simulink model "vr_octavia_mirror"  (Simulink 7.7)
settings: Solver=VariableStepDiscrete  StartTime=0.0  StopTime=111.56  RelTol=1e-3
PostLoadFcn:
  | load octavia_testlap
libraries: vrlib x26, simulink x1
Description:
  | Vehicle Dynamics Visualization with Live Rear Mirror Image
  | 
  | This example extends the vr_octavia example to demonstrate the capability
  | of the VR Sink block to process video stream on input.
  | 
  | In the virtual world, a VRML97 PixelTexture texture map is defined
  | at the place of the vehicle left rear mirror. 2D image from a viewpoint placed
  | at the same position (looking backwards) is mirrored and looped back into
  | the same virtual world and projected on the rear mirror glass - creating
  | an impression of live reflection.
  | 
  | Texture image can have different formats (corresponding to the available
  | SFImage definitions according to the VRML97 standard), in this case
  | we use an RGB image that has the same format as the output from the
  | VR to Video block. Note that in the VRML file associated with the scene,
  | it is possible to define only a trivial texture (in our case, a 4x4 pixel
  | checkerboard) that will get resized during simulation according to the current
  | size of the signal on the input.
settings Model: Creator=Danek  LastModifiedBy=Danek  ExtModeArmWhenConnect=off  BufferReuse=off
settings SolverCC: InsertRTBMode=Auto
settings DataIOCC: SignalLoggingName=sigsOut
settings OptimizationCC: BooleanDataType=off  InlineInvariantSignals=on  OptimizeBlockIOStorage=off  BufferReuse=off  ExpressionFolding=off  LocalBlockOutputs=off  InitFltsAndDblsToZero=on
settings DebuggingCC: CheckExecutionContextPreStartOutputMsg=on  CheckExecutionContextRuntimeOutputMsg=on  SignalResolutionControl=TryResolveAllWithWarning  SolverPrmCheckMsg=none  MultiTaskDSMMsg=warning  MultiTaskCondExecSysMsg=none  StrictBusMsg=None
settings RTWCC: RetainRTWFile=on  ProcessScript=grt_make_rtw_hook  IncludeERTFirstTime=on
settings GRTTargetCC: TargetFcnLib=ansi_tfl_tmw.mat

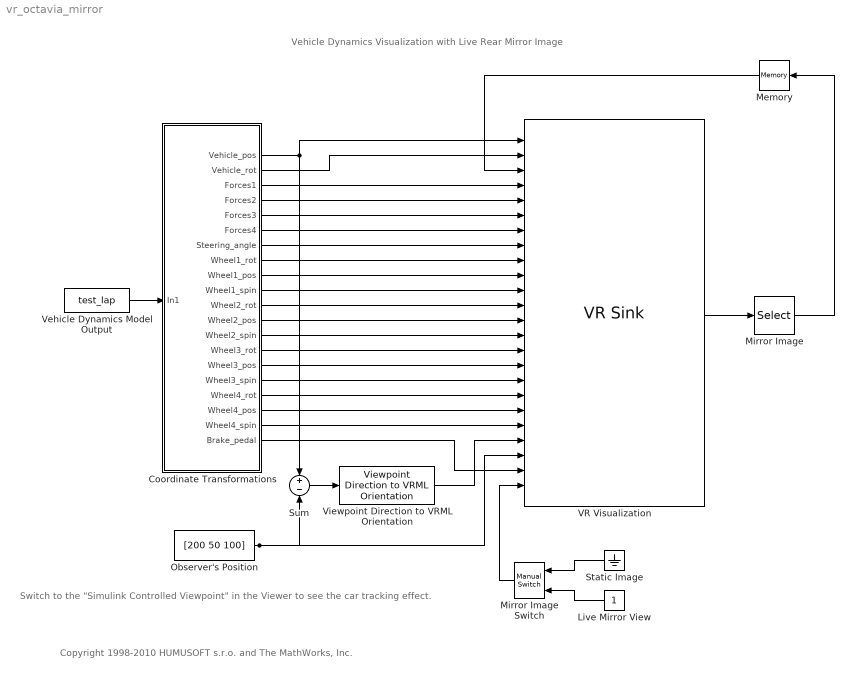
== system vr_octavia_mirror ==
  note: Vehicle Dynamics Visualization with Live Rear Mirror Image
  note: Switch to the "Simulink Controlled Viewpoint"
      | in the Viewer to see the car tracking effect.
  note: Copyright 1998-2010 HUMUSOFT s.r.o. and The MathWorks, Inc.
  Coordinate Transformations : Subsystem
  Live Mirror View : Constant
  Memory : Memory
  Mirror Image : Selector  NumberOfDimensions=3  InputPortWidth=3  IndexOptions=Select all,Index vector (dialog),Select all  Indices=200:-1:1,160:-1:1,1  OutputSizes=1,1,1
  Mirror Image Switch : simulink/Signal Routing/Manual Switch  SystemSampleTime=-1  sw=0  action=0  varsize=off
  Observer's Position : Constant  Value=[200 50 100]
  Static Image : Ground
  Sum : Sum  Inputs=+-
  VR Visualization : vrlib/VR Sink  InstantiateOnLoad=on  SampleTime=0.1  ViewEnable=on  RemoteChange=off  RemoteView=on  FieldsWritten=Vehicle_pos_Car1.translation.3.1.1.double#Vehicle_rot_Car1.rotation.4.1.1.double#Mirror_Image_Car1.image.-1.-1.-1.uint8#Force1_Car1.scale.3.1.1.double#Force2_Car1.scale.3.1.1.double#Force3_Car1.scale.3.1.1.double#Force4_Car1.scale.3.1.1.double#SteeringWheelAngle1_Car1.rotation.4.1.1.double#WheelFL_Car1.rotation.4.1.1.double#WheelFL_Car1.translation.3.1.1.double#WheelSpinFL_Car1.rotation.4.1.1.double#WheelFR_Car1.rotation.4.1.1.double#WheelFR_Car1.translation.3.1.1.double#WheelSpinFR_Car1.rotation.4.1.1.double#WheelRL_Car1.rotation.4.1.1.double#WheelRL_Car1.translation.3.1.1.double#WheelSpinRL_Car1.rotation.4.1.1.double#WheelRR_Car1.rotation.4.1.1.double#WheelRR_Car1.translation.3.1.1.double#WheelSpinRR_Car1.rotation.4.1.1.double#FlyingCamera.orientation.4.1.1.double#FlyingCamera.position.3.1.1.double#Brake_Switch_Car1.whichChoice.1.1.1.double#Mirror_Switch_Car1.whichChoice.1.1.1.double  WorldFileName=octavia_scene.wrl  WorldDescription=Vehicle Dynamics Visualization - Skoda Octavia  AutoView=on  VideoDimensions=[100 160]  FigureProperties="{'Position', 'Name', 'Viewpoint', 'CameraBound', 'CameraDirection', 'CameraPosition', 'CameraUpVector', 'ZoomFactor', 'Antialiasing', 'Headlight', 'Lighting', 'NavPanel', 'StatusBar', 'ToolBar', 'Textures', 'Transparency', 'Wireframe', 'NavZones', 'NavMode', 'NavSpeed', 'Record2DCompressMethod', 'Record2DCompressQuality', 'Record2D', 'Record2DFileName', 'Record2DFPS'; [1.9000000000000000e+001  8.9000000000000000e+001  5.7600000000000000e+002  3.8000000000000000e+002], 'Vehicle Dynamics Visualization - Skoda Octavia', 'Driver''s View - Car1', 'on', [0.0000000000000000e+000  0.0000000000000000e+000 -1.0000000000000000e+000], [0.0000000000000000e+000  0.0000000000000000e+000  0.0000000000000000e+000], [0.0000000000000000e+000  1.0000000000000000e+000  0.0000000000000000e+000], [1.0000000000000000e+000], 'on', 'off', 'on', 'halfbar', 'on', 'on', 'on', 'on', 'off', 'off', 'walk', 'normal', 'auto', [7.5000000000000000e+001], 'off', '%f_anim_%n.avi', [1.5000000000000000e+001]; [6.0000000000000000e+002  6.0000000000000000e+001  1.6000000000000000e+002  1.0000000000000000e+002], 'Vehicle Dynamics Visualization - Skoda Octavia', 'Car1 - View from Above Ahead - Rot', 'on', [5.8249750547694490e-001  5.2158739247318453e-001 -6.2341258258569376e-001], [8.0602203932287431e-001  7.6180911249256611e-001 -8.8299607282409376e+000], [6.8248003830141860e-002  7.3287086238403754e-001  6.7693611887805349e-001], [7.5131480090157765e-001], 'on', 'off', 'on', 'none', 'off', 'off', 'on', 'on', 'off', 'off', 'walk', 'veryslow', 'auto', [7.5000000000000000e+001], 'off', '***video***', [1.5000000000000000e+001]}"
  Vehicle Dynamics Model Output : FromWorkspace  VariableName=test_lap  SampleTime=0.04  OutputAfterFinalValue=Holding final value
  Viewpoint Direction to VRML Orientation : vrlib/Utilities/Viewpoint Direction to VRML Orientation  SystemSampleTime=-1
  wires:
  Vehicle Dynamics Model Output/1 -> Coordinate Transformations/1(In1)
  Sum/1 -> Viewpoint Direction to VRML Orientation/1
  Observer's Position/1 -> Sum/2, VR Visualization/22
  VR Visualization/1 -> Mirror Image/1
  Mirror Image/1 -> Memory/1
  Coordinate Transformations/1(Vehicle_pos) -> Sum/1, VR Visualization/1
  Static Image/1 -> Mirror Image Switch/1
  Live Mirror View/1 -> Mirror Image Switch/2
  Coordinate Transformations/2(Vehicle_rot) -> VR Visualization/2
  Memory/1 -> VR Visualization/3
  Coordinate Transformations/3(Forces1) -> VR Visualization/4
  Coordinate Transformations/4(Forces2) -> VR Visualization/5
  Coordinate Transformations/5(Forces3) -> VR Visualization/6
  Coordinate Transformations/6(Forces4) -> VR Visualization/7
  Coordinate Transformations/7(Steering_angle) -> VR Visualization/8
  Coordinate Transformations/8(Wheel1_rot) -> VR Visualization/9
  Coordinate Transformations/9(Wheel1_pos) -> VR Visualization/10
  Coordinate Transformations/10(Wheel1_spin) -> VR Visualization/11
  Coordinate Transformations/11(Wheel2_rot) -> VR Visualization/12
  Coordinate Transformations/12(Wheel2_pos) -> VR Visualization/13
  Coordinate Transformations/13(Wheel2_spin) -> VR Visualization/14
  Coordinate Transformations/14(Wheel3_rot) -> VR Visualization/15
  Coordinate Transformations/15(Wheel3_pos) -> VR Visualization/16
  Coordinate Transformations/16(Wheel3_spin) -> VR Visualization/17
  Coordinate Transformations/17(Wheel4_rot) -> VR Visualization/18
  Coordinate Transformations/18(Wheel4_pos) -> VR Visualization/19
  Coordinate Transformations/19(Wheel4_spin) -> VR Visualization/20
  Viewpoint Direction to VRML Orientation/1 -> VR Visualization/21
  Coordinate Transformations/20(Brake_pedal) -> VR Visualization/23
  Mirror Image Switch/1 -> VR Visualization/24

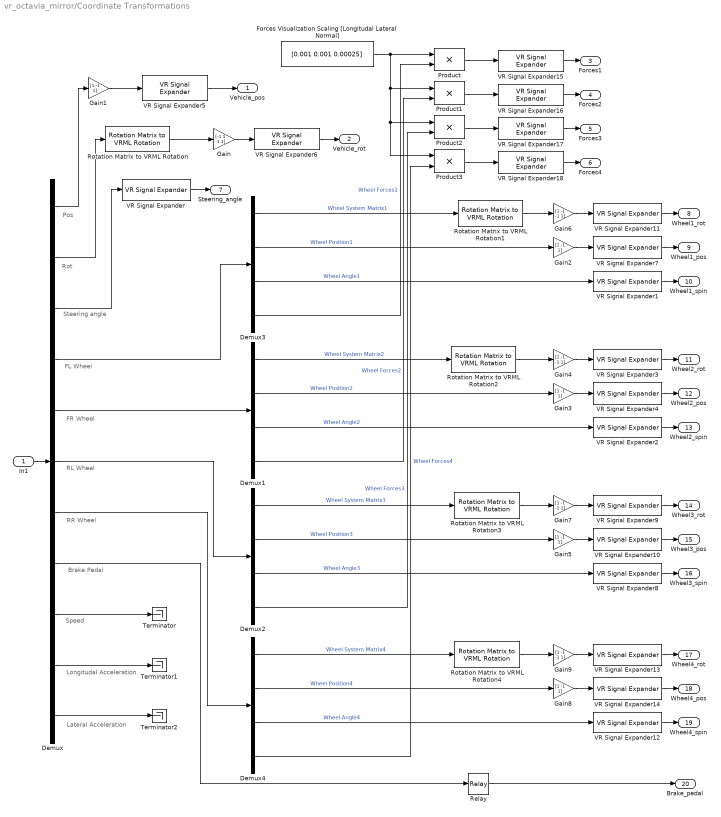
== system vr_octavia_mirror/Coordinate Transformations ==
  note: Steering angle
  note: FL Wheel
  note: FR Wheel
  note: RL Wheel
  note: RR Wheel
  note: Brake Pedal
  note: Pos
  note: Rot
  note: Speed
  note: Longitudal Acceleration
  note: Lateral Acceleration
  In1 : Inport
  Demux : Demux  Outputs=[3,9,1,16,16,16,16,1,1,1,1]
  Demux{1..4} (4 alike) : Demux  Outputs=[9,3,1,3]
  Forces Visualization Scaling [Longitudal Lateral Normal] : Constant  Value=[0.001 0.001 0.00025]
  Gain : Gain  Gain=[-1 1 -1 1]  SaturateOnIntegerOverflow=on  OutDataTypeStr=Inherit: Same as input  ParamDataTypeStr=Inherit: Same as input
  Gain{1..3,5,8} (5 alike) : Gain  Gain=[1 -1 1]  SaturateOnIntegerOverflow=on  OutDataTypeStr=Inherit: Same as input  ParamDataTypeStr=Inherit: Same as input
  Gain{4,6..7,9} (4 alike) : Gain  Gain=[1 -1 -1 1]  SaturateOnIntegerOverflow=on  OutDataTypeStr=Inherit: Same as input  ParamDataTypeStr=Inherit: Same as input
  Product{,1..3} (4 alike) : Product  SaturateOnIntegerOverflow=on  OutDataTypeStr=Inherit: Same as first input
  Relay : Relay
  Rotation Matrix to VRML Rotation{,1..4} (5 alike) : vrlib/Utilities/Rotation Matrix to VRML Rotation  SystemSampleTime=-1  maxzero=1e-12
  Terminator : Terminator
  Terminator1 : Terminator
  Terminator2 : Terminator
  VR Signal Expander{,1..2,8,12} (5 alike) : vrlib/VR Signal Expander  SystemSampleTime=-1  outwidth=4  outidx=[4]
  VR Signal Expander{4,7,10,14} (4 alike) : vrlib/VR Signal Expander  SystemSampleTime=-1  outwidth=3  outidx=[1 3 2 ]
  VR Signal Expander{3,6,9,11,13} (5 alike) : vrlib/VR Signal Expander  SystemSampleTime=-1  outwidth=4  outidx=[1 3 2 4]
  VR Signal Expander{5,15..18} (5 alike) : vrlib/VR Signal Expander  SystemSampleTime=-1  outwidth=3  outidx=[1 3 2]
  Vehicle_pos : Outport
  Vehicle_rot : Outport  Port=2
  Forces1 : Outport  Port=3
  Forces2 : Outport  Port=4
  Forces3 : Outport  Port=5
  Forces4 : Outport  Port=6
  Steering_angle : Outport  Port=7
  Wheel1_rot : Outport  Port=8
  Wheel1_pos : Outport  Port=9
  Wheel1_spin : Outport  Port=10
  Wheel2_rot : Outport  Port=11
  Wheel2_pos : Outport  Port=12
  Wheel2_spin : Outport  Port=13
  Wheel3_rot : Outport  Port=14
  Wheel3_pos : Outport  Port=15
  Wheel3_spin : Outport  Port=16
  Wheel4_rot : Outport  Port=17
  Wheel4_pos : Outport  Port=18
  Wheel4_spin : Outport  Port=19
  Brake_pedal : Outport  Port=20
  wires:
  Gain1/1 -> VR Signal Expander5/1
  Rotation Matrix to VRML Rotation/1 -> Gain/1
  Gain/1 -> VR Signal Expander6/1
  Gain6/1 -> VR Signal Expander11/1
  Gain2/1 -> VR Signal Expander7/1
  Demux3/1 -> Rotation Matrix to VRML Rotation1/1  "Wheel System Matrix1"
  Demux3/2 -> Gain2/1  "Wheel Position1"
  Demux3/3 -> VR Signal Expander1/1  "Wheel Angle1"
  Gain4/1 -> VR Signal Expander3/1
  Rotation Matrix to VRML Rotation2/1 -> Gain4/1
  Gain3/1 -> VR Signal Expander4/1
  Demux1/1 -> Rotation Matrix to VRML Rotation2/1  "Wheel System Matrix2"
  Demux1/2 -> Gain3/1  "Wheel Position2"
  Demux1/3 -> VR Signal Expander2/1  "Wheel Angle2"
  Gain7/1 -> VR Signal Expander9/1
  Rotation Matrix to VRML Rotation3/1 -> Gain7/1
  Demux2/4 -> Product2/2  "Wheel Forces3"
  Gain5/1 -> VR Signal Expander10/1
  Demux2/1 -> Rotation Matrix to VRML Rotation3/1  "Wheel System Matrix3"
  Demux2/2 -> Gain5/1  "Wheel Position3"
  Demux2/3 -> VR Signal Expander8/1  "Wheel Angle3"
  Gain9/1 -> VR Signal Expander13/1
  Rotation Matrix to VRML Rotation4/1 -> Gain9/1
  Demux4/4 -> Product3/2  "Wheel Forces4"
  Gain8/1 -> VR Signal Expander14/1
  Demux4/1 -> Rotation Matrix to VRML Rotation4/1  "Wheel System Matrix4"
  Demux4/2 -> Gain8/1  "Wheel Position4"
  Demux4/3 -> VR Signal Expander12/1  "Wheel Angle4"
  VR Signal Expander5/1 -> Vehicle_pos/1
  Demux3/4 -> Product/2  "Wheel Forces1"
  Demux1/4 -> Product1/2  "Wheel Forces2"
  Product/1 -> VR Signal Expander15/1
  Product1/1 -> VR Signal Expander16/1
  Product2/1 -> VR Signal Expander17/1
  Product3/1 -> VR Signal Expander18/1
  VR Signal Expander6/1 -> Vehicle_rot/1
  VR Signal Expander15/1 -> Forces1/1
  VR Signal Expander16/1 -> Forces2/1
  VR Signal Expander17/1 -> Forces3/1
  VR Signal Expander18/1 -> Forces4/1
  VR Signal Expander/1 -> Steering_angle/1
  VR Signal Expander11/1 -> Wheel1_rot/1
  In1/1 -> Demux/1
  VR Signal Expander7/1 -> Wheel1_pos/1
  VR Signal Expander1/1 -> Wheel1_spin/1
  VR Signal Expander3/1 -> Wheel2_rot/1
  VR Signal Expander4/1 -> Wheel2_pos/1
  VR Signal Expander2/1 -> Wheel2_spin/1
  VR Signal Expander9/1 -> Wheel3_rot/1
  VR Signal Expander10/1 -> Wheel3_pos/1
  VR Signal Expander8/1 -> Wheel3_spin/1
  VR Signal Expander13/1 -> Wheel4_rot/1
  VR Signal Expander14/1 -> Wheel4_pos/1
  VR Signal Expander12/1 -> Wheel4_spin/1
  Demux/8 -> Relay/1
  Relay/1 -> Brake_pedal/1
  Demux/1 -> Gain1/1
  Demux/2 -> Rotation Matrix to VRML Rotation/1
  Demux/3 -> VR Signal Expander/1
  Demux/4 -> Demux3/1
  Demux/5 -> Demux1/1
  Demux/6 -> Demux2/1
  Demux/7 -> Demux4/1
  Forces Visualization Scaling [Longitudal Lateral Normal]/1 -> Product/1, Product1/1, Product2/1, Product3/1
  Rotation Matrix to VRML Rotation1/1 -> Gain6/1
  Demux/9 -> Terminator/1
  Demux/10 -> Terminator1/1
  Demux/11 -> Terminator2/1
